simulink model "PitchControl_OpenLoop"  (R2024b)
settings: Solver=VariableStepAuto  StartTime=0.0  StopTime=10.0  RelTol=1e-3
settings Model: Creator=Arghya  LastModifiedBy=Arghya

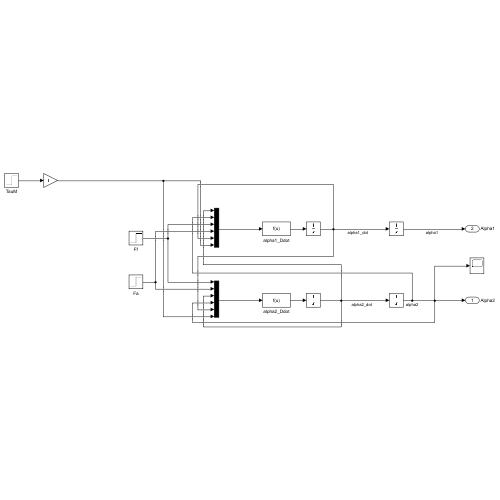
[thumbnail: Simulink's stored preview of the top-level diagram]
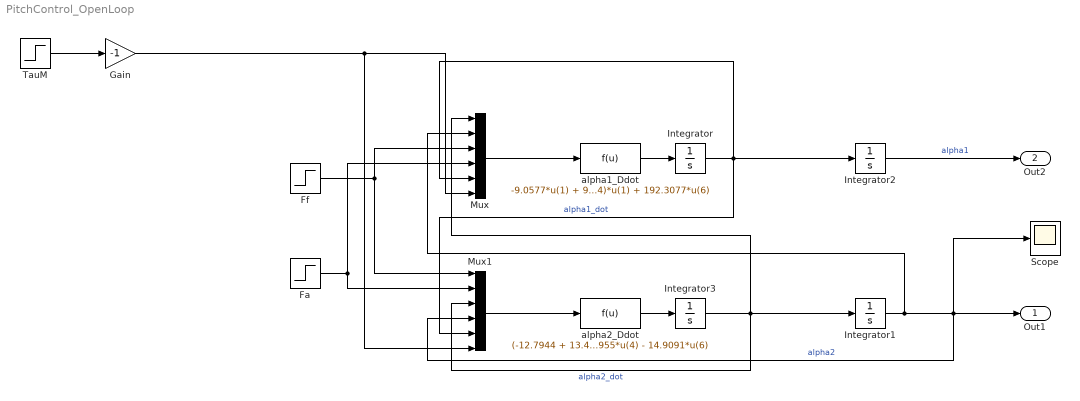
== system PitchControl_OpenLoop ==
  Fa : Step  SampleTime=0.2
  Ff : Step  SampleTime=0.2
  Gain : Gain  Gain=-1
  Integrator : Integrator  UpperSaturationLimit=pi  LowerSaturationLimit=0  ContinuousStateAttributes="\"alpha1_dot\""
  Integrator1 : Integrator  ContinuousStateAttributes="\"alpha2\""
  Integrator2 : Integrator  ContinuousStateAttributes="\"alpha1\""
  Integrator3 : Integrator  UpperSaturationLimit=pi/2  LowerSaturationLimit=-pi/2  ContinuousStateAttributes="\"alpha2_dot\""
  Mux : Mux  Inputs=6
  Mux1 : Mux  Inputs=6
  Scope : Scope
  TauM : Step  SampleTime=0.2
  alpha1_Ddot : Fcn  Expr=-9.0577*u(1) + 9.0577*u(2)*u(1)*u(1) - 192.3077*(u(3)+u(4))*u(5) + 192.3077*u(4)*u(1) + 192.3077*u(6)
  alpha2_Ddot : Fcn  Expr=(-12.7944 + 13.4268*u(1) + 11.944*u(2))*u(3) - 0.6324*u(4)*u(3)*u(3) + 1.4824*u(5) + 12.1955*u(4) - 14.9091*u(6)
  Out1 : Outport  SignalName=Alpha2
  Out2 : Outport  Port=2  SignalName=Alpha1
  wires:
  Integrator/1 -> Mux1/5, Mux/5, Integrator2/1  "alpha1_dot"
  alpha1_Ddot/1 -> Integrator/1
  Integrator3/1 -> Mux/1, Mux1/3, Integrator1/1  "alpha2_dot"
  alpha2_Ddot/1 -> Integrator3/1
  Integrator2/1 -> Out2/1  "alpha1"
  Integrator1/1 -> Mux/2, Scope/1, Mux1/4, Out1/1  "alpha2"
  Ff/1 -> Mux/3, Mux1/1
  Fa/1 -> Mux1/2, Mux/4
  Mux/1 -> alpha1_Ddot/1
  Mux1/1 -> alpha2_Ddot/1
  TauM/1 -> Gain/1
  Gain/1 -> Mux1/6, Mux/6
